simulink model "k1visitmxp"  (Simulink 8.8)
settings: Solver=ode45  StartTime=0.0  StopTime=10.0  RelTol=1e-3  EnableMultiTasking=on
libraries: cdsIPCx x26, cdsCDI64 x6, cdsCDO64 x6, BIO_CD_DECODE_MASTER x6, BIO_CD_ENCODE_MASTER x5, CHK_DIO x5, dac x3, cdsBit2Word x2, cdsAdcx0 x1, cdsAdcx1 x1, TYPEA_MASTER x1, cdsEpicsOut x1
settings Model: SuppressorTable=22 serialization::archive 11 0 3 0 0 0 11 0  Creator=controls  LastModifiedBy=controls
settings DataIOCC: SignalLoggingSaveFormat=Dataset
settings DebuggingCC: UnderspecifiedInitializationDetection=Simplified  MergeDetectMultiDrivingBlocksExec=error  FcnCallInpInsideContextMsg=error  AllowSymbolicDim=off  StateNameClashWarn=none
settings GRTTargetCC: CombineOutputUpdateFcns=on  GRTInterface=off

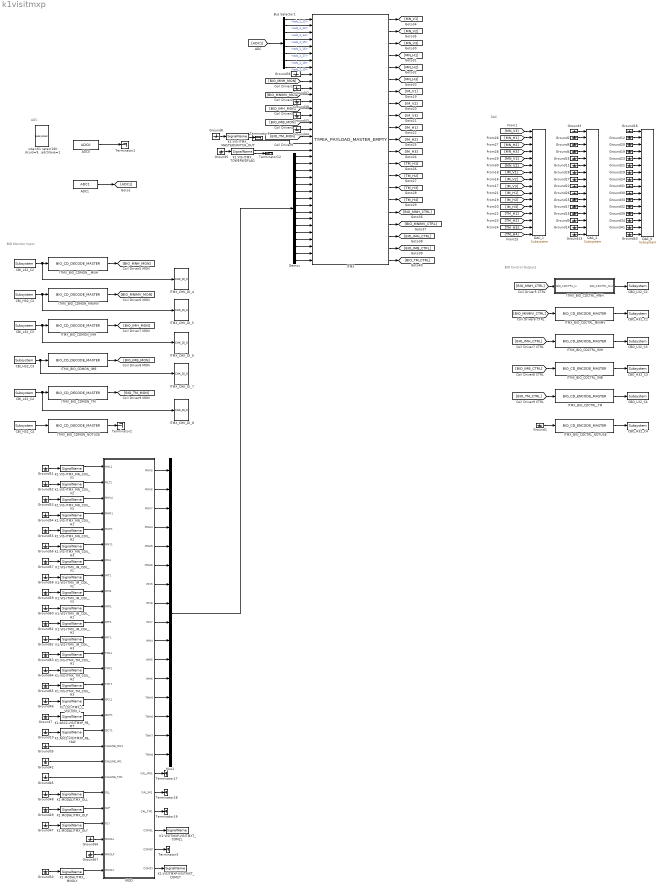
== system k1visitmxp ==
  note: BIO Monitor Input
  note: BIO Control Outputs
  note: DAC
  note: ADC
  ADC0 : cdsAdcx0/ADC0  Tag=cdsAdc  Description=|
      | type-GSC_16AI64SSA
      | card_num=0
      settings: AttributesFormatString=%<Description>\n%<Tag>
  ADC1 : cdsAdcx1/ADC1  Tag=cdsAdc  Description=|
      | type-GSC_16AI64SSA
      | card_num=1
      settings: AttributesFormatString=%<Description>\n%<Tag>
  Bus Selector1 : BusSelector  OutputSignals=adc_1_12,adc_1_13,adc_1_14,adc_1_15,adc_1_16,adc_1_17,adc_1_18,adc_1_19
  CBI_H32_C2 : cdsCDI64/Subsystem  Tag=cdsCDI64  Description=card_num=5
      settings: AttributesFormatString=%<Tag>\n%<Description>
  CBI_H32_C3 : cdsCDI64/Subsystem  Tag=cdsCDI64  Description=card_num=7
      settings: AttributesFormatString=%<Tag>\n%<Description>
  CBI_H32_C4 : cdsCDI64/Subsystem  Tag=cdsCDI64  Description=card_num=9
      settings: AttributesFormatString=%<Tag>\n%<Description>
  CBI_L32_C2 : cdsCDI64/Subsystem  Tag=cdsCDI64  Description=card_num=4
      settings: AttributesFormatString=%<Tag>\n%<Description>
  CBI_L32_C3 : cdsCDI64/Subsystem  Tag=cdsCDI64  Description=card_num=6
      settings: AttributesFormatString=%<Tag>\n%<Description>
  CBI_L32_C4 : cdsCDI64/Subsystem  Tag=cdsCDI64  Description=card_num=8
      settings: AttributesFormatString=%<Tag>\n%<Description>
  CBO_H32_C2 : cdsCDO64/Subsystem  Tag=cdsCDO64  Description=card_num=5
      settings: AttributesFormatString=%<Tag>\n%<Description>
  CBO_H32_C3 : cdsCDO64/Subsystem  Tag=cdsCDO64  Description=card_num=7
      settings: AttributesFormatString=%<Tag>\n%<Description>
  CBO_H32_C4 : cdsCDO64/Subsystem  Tag=cdsCDO64  Description=card_num=9
      settings: AttributesFormatString=%<Tag>\n%<Description>
  CBO_L32_C2 : cdsCDO64/Subsystem  Tag=cdsCDO64  Description=card_num=4
      settings: AttributesFormatString=%<Tag>\n%<Description>
  CBO_L32_C3 : cdsCDO64/Subsystem  Tag=cdsCDO64  Description=card_num=6
      settings: AttributesFormatString=%<Tag>\n%<Description>
  CBO_L32_C4 : cdsCDO64/Subsystem  Tag=cdsCDO64  Description=card_num=8
      settings: AttributesFormatString=%<Tag>\n%<Description>
  DAC_0 : dac/Subsystem  Description=|
      | type=GSC_16AO16,
      | card_num=0
      settings: AttributesFormatString=%<Description>
  DAC_1 : dac/Subsystem  Description=|
      | type=GSC_16AO16,
      | card_num=1
      settings: AttributesFormatString=%<Description>
  DAC_2 : dac/Subsystem  Description=|
      | type=GSC_16AO16,
      | card_num=2
      settings: AttributesFormatString=%<Description>
  Demux : Demux  Outputs=16
  Ground{1..67} (67 alike) : Ground
  ITMX : TYPEA_MASTER/TYPEA_PAYLOAD_MASTER_EMPTY
  ITMX_BIO_CDCTRL_IMB : BIO_CD_ENCODE_MASTER/BIO_CD_ENCODE_MASTER
  ITMX_BIO_CDCTRL_IMH : BIO_CD_ENCODE_MASTER/BIO_CD_ENCODE_MASTER
  ITMX_BIO_CDCTRL_MNH : Subsystem
  ITMX_BIO_CDCTRL_MNIMV : BIO_CD_ENCODE_MASTER/BIO_CD_ENCODE_MASTER
  ITMX_BIO_CDCTRL_NOTUSE : BIO_CD_ENCODE_MASTER/BIO_CD_ENCODE_MASTER
  ITMX_BIO_CDCTRL_TM : BIO_CD_ENCODE_MASTER/BIO_CD_ENCODE_MASTER
  ITMX_BIO_CDMON_IMB : BIO_CD_DECODE_MASTER/BIO_CD_DECODE_MASTER
  ITMX_BIO_CDMON_IMH : BIO_CD_DECODE_MASTER/BIO_CD_DECODE_MASTER
  ITMX_BIO_CDMON_MNIMV : BIO_CD_DECODE_MASTER/BIO_CD_DECODE_MASTER
  ITMX_BIO_CDMON_NOTUSE : BIO_CD_DECODE_MASTER/BIO_CD_DECODE_MASTER
  ITMX_BIO_CDMON_TM : BIO_CD_DECODE_MASTER/BIO_CD_DECODE_MASTER
  ITMX_BIO_CDMON__MNH : BIO_CD_DECODE_MASTER/BIO_CD_DECODE_MASTER
  ITMX_CHK_DI_{4..8} (5 alike) : CHK_DIO/CHK_DI_0
  K1:ASC2-VISITMXP_FB_PIT : cdsIPCx/SignalName  Tag=cdsIPCx_RFM  Description=card=0
      settings: AttributesFormatString=%<Description>\n%<Tag>
  K1:ASC2-VISITMXP_FB_YAW : cdsIPCx/SignalName  Tag=cdsIPCx_RFM  Description=card=0
      settings: AttributesFormatString=%<Description>\n%<Tag>
  K1:LSC-ITMX_L_VISITMX_L : cdsIPCx/SignalName  Tag=cdsIPCx_RFM  Description=card=0
      settings: AttributesFormatString=%<Description>\n%<Tag>
  K1:MODALITMX_MNOLY : cdsIPCx/SignalName  Tag=cdsIPCx_SHMEM  Description=Inter-Process Communication via Shared memory.
      settings: AttributesFormatString=%<Tag>
  K1:MODALITMX_OLL : cdsIPCx/SignalName  Tag=cdsIPCx_SHMEM  Description=Inter-Process Communication via Shared memory.
      settings: AttributesFormatString=%<Tag>
  K1:MODALITMX_OLP : cdsIPCx/SignalName  Tag=cdsIPCx_SHMEM  Description=Inter-Process Communication via Shared memory.
      settings: AttributesFormatString=%<Tag>
  K1:MODALITMX_OLY : cdsIPCx/SignalName  Tag=cdsIPCx_SHMEM  Description=Inter-Process Communication via Shared memory.
      settings: AttributesFormatString=%<Tag>
  K1:VIS-ITMX_IM_COIL_H1 : cdsIPCx/SignalName  Tag=cdsIPCx_SHMEM  Description=Inter-Process Communication via Shared memory.
      settings: AttributesFormatString=%<Tag>
  K1:VIS-ITMX_IM_COIL_H2 : cdsIPCx/SignalName  Tag=cdsIPCx_SHMEM  Description=Inter-Process Communication via Shared memory.
      settings: AttributesFormatString=%<Tag>
  K1:VIS-ITMX_IM_COIL_H3 : cdsIPCx/SignalName  Tag=cdsIPCx_SHMEM  Description=Inter-Process Communication via Shared memory.
      settings: AttributesFormatString=%<Tag>
  K1:VIS-ITMX_IM_COIL_V1 : cdsIPCx/SignalName  Tag=cdsIPCx_SHMEM  Description=Inter-Process Communication via Shared memory.
      settings: AttributesFormatString=%<Tag>
  K1:VIS-ITMX_IM_COIL_V2 : cdsIPCx/SignalName  Tag=cdsIPCx_SHMEM  Description=Inter-Process Communication via Shared memory.
      settings: AttributesFormatString=%<Tag>
  K1:VIS-ITMX_IM_COIL_V3 : cdsIPCx/SignalName  Tag=cdsIPCx_SHMEM  Description=Inter-Process Communication via Shared memory.
      settings: AttributesFormatString=%<Tag>
  K1:VIS-ITMX_MASTERSWITCH_OUT : cdsIPCx/SignalName  Tag=cdsIPCx_SHMEM  Description=Inter-Process Communication via Shared memory.
      settings: AttributesFormatString=%<Tag>
  K1:VIS-ITMX_MN_COIL_H1 : cdsIPCx/SignalName  Tag=cdsIPCx_SHMEM  Description=Inter-Process Communication via Shared memory.
      settings: AttributesFormatString=%<Tag>
  K1:VIS-ITMX_MN_COIL_H2 : cdsIPCx/SignalName  Tag=cdsIPCx_SHMEM  Description=Inter-Process Communication via Shared memory.
      settings: AttributesFormatString=%<Tag>
  K1:VIS-ITMX_MN_COIL_H3 : cdsIPCx/SignalName  Tag=cdsIPCx_SHMEM  Description=Inter-Process Communication via Shared memory.
      settings: AttributesFormatString=%<Tag>
  K1:VIS-ITMX_MN_COIL_V1 : cdsIPCx/SignalName  Tag=cdsIPCx_SHMEM  Description=Inter-Process Communication via Shared memory.
      settings: AttributesFormatString=%<Tag>
  K1:VIS-ITMX_MN_COIL_V2 : cdsIPCx/SignalName  Tag=cdsIPCx_SHMEM  Description=Inter-Process Communication via Shared memory.
      settings: AttributesFormatString=%<Tag>
  K1:VIS-ITMX_MN_COIL_V3 : cdsIPCx/SignalName  Tag=cdsIPCx_SHMEM  Description=Inter-Process Communication via Shared memory.
      settings: AttributesFormatString=%<Tag>
  K1:VIS-ITMX_TM_COIL_H1 : cdsIPCx/SignalName  Tag=cdsIPCx_SHMEM  Description=Inter-Process Communication via Shared memory.
      settings: AttributesFormatString=%<Tag>
  K1:VIS-ITMX_TM_COIL_H2 : cdsIPCx/SignalName  Tag=cdsIPCx_SHMEM  Description=Inter-Process Communication via Shared memory.
      settings: AttributesFormatString=%<Tag>
  K1:VIS-ITMX_TM_COIL_H3 : cdsIPCx/SignalName  Tag=cdsIPCx_SHMEM  Description=Inter-Process Communication via Shared memory.
      settings: AttributesFormatString=%<Tag>
  K1:VIS-ITMX_TOWERWDFLAG : cdsIPCx/SignalName  Tag=cdsIPCx_SHMEM  Description=Inter-Process Communication via Shared memory.
      settings: AttributesFormatString=%<Tag>
  K1:VISITMXP-VISITMXT_COM2L : cdsIPCx/SignalName  Tag=cdsIPCx_SHMEM  Description=Inter-Process Communication via Shared memory.
      settings: AttributesFormatString=%<Tag>
  K1:VISITMXP-VISITMXT_COM2Y : cdsIPCx/SignalName  Tag=cdsIPCx_SHMEM  Description=Inter-Process Communication via Shared memory.
      settings: AttributesFormatString=%<Tag>
  MOD : Subsystem  Tag=top_names
  Mux1 : Mux  Inputs=16
  Terminator{1..3,9,12,17..19} (8 alike) : Terminator
  site=K1 rate=16K dcuid=93 host=k1ix1 specific_cpu=3 adcSlave=1 : cdsParameters/Subsystem  Tag=cdsParameters  Description=|
      | Purpose:                                                                                                                                                                                                                                
      | Provide system parameters to the FE code generator to properly configure the generated EPICS names, rep rate of the FE controller, and the Data Acquisition node ID for proper storage of data from this FE controller.                 
      |                                                                                                                                                                                                                                         
      | Useage:                                                                                                                                                                                                                                 
      | The part NAME field is used to identify the FE parameters. It must be of the form:                                                                                                                                                      
      | site=                                                                                                                                                                                                                                   
      | rate=                                                                                                                                                                                                                                   
      | dcuid=                                                                                                                                                                                                                                  
      |                                                                                                                                                                                                                                         
      | Where:                                                                                                                                                                                                                                  
      | site= argument may be H1, H2, L1, M1, G1, either as a single argument or multiple, for example site=H1,H2. These are the only names allowed. These will become the first two characters of all EPICS and signal names (for example G1:).
      |                                                                                                                                                                                                                                         
      | rate= may be 2K, 16K, 32K, or 64K                                                                                                                                                                                                       
      |                                                                                                                                                                                                                                         
      | dcuid= is site specific ie it must be unique at each site.
      settings: AttributesFormatString=%<Tag>
  wires:
  ADC1/1 -> [ADC1]
  [MN_V3] -> DAC_1/1
  [MN_H1] -> DAC_1/2
  [MN_H2] -> DAC_1/3
  [MN_H3] -> DAC_1/4
  [MN_V1] -> DAC_1/5
  [MN_V2] -> DAC_1/6
  [IM_V1] -> DAC_1/7
  [IM_V2] -> DAC_1/8
  [IM_V3] -> DAC_1/9
  [IM_H1] -> DAC_1/10
  [TM_H1] -> DAC_1/13
  [TM_H4] -> DAC_1/16
  [TM_H3] -> DAC_1/15
  [TM_H2] -> DAC_1/14
  [IM_H2] -> DAC_1/11
  [IM_H3] -> DAC_1/12
  [BIO_MNH_CTRL] -> ITMX_BIO_CDCTRL_MNH/1(BIO_CDCTRL_In)
  ITMX_BIO_CDCTRL_MNH/1(DIO_CDCTRL_Out) -> CBO_L32_C2/1
  [BIO_MNIMV_CTRL] -> ITMX_BIO_CDCTRL_MNIMV/1
  ITMX_BIO_CDCTRL_MNIMV/1 -> CBO_H32_C2/1
  [BIO_IMH_CTRL] -> ITMX_BIO_CDCTRL_IMH/1
  ITMX_BIO_CDCTRL_IMH/1 -> CBO_L32_C3/1
  [BIO_IMB_CTRL] -> ITMX_BIO_CDCTRL_IMB/1
  ITMX_BIO_CDCTRL_IMB/1 -> CBO_H32_C3/1
  [BIO_TM_CTRL] -> ITMX_BIO_CDCTRL_TM/1
  ITMX_BIO_CDCTRL_TM/1 -> CBO_L32_C4/1
  Ground1/1 -> ITMX_BIO_CDCTRL_NOTUSE/1
  ITMX_BIO_CDCTRL_NOTUSE/1 -> CBO_H32_C4/1
  CBI_L32_C2/1 -> ITMX_CHK_DI_4/1, ITMX_BIO_CDMON__MNH/1
  ITMX_BIO_CDMON__MNH/1 -> [BIO_MNH_MON]
  CBI_H32_C2/1 -> ITMX_CHK_DI_5/1, ITMX_BIO_CDMON_MNIMV/1
  ITMX_BIO_CDMON_MNIMV/1 -> [BIO_MNIMV_MON]
  CBI_L32_C3/1 -> ITMX_CHK_DI_6/1, ITMX_BIO_CDMON_IMH/1
  ITMX_BIO_CDMON_IMH/1 -> [BIO_IMH_MON]
  ITMX_BIO_CDMON_IMB/1 -> [BIO_IMB_MON]
  CBI_L32_C4/1 -> ITMX_CHK_DI_8/1, ITMX_BIO_CDMON_TM/1
  ITMX_BIO_CDMON_TM/1 -> [BIO_TM_MON]
  CBI_H32_C4/1 -> ITMX_BIO_CDMON_NOTUSE/1
  ITMX_BIO_CDMON_NOTUSE/1 -> Terminator2/1
  Ground3/1 -> DAC_2/1
  Ground2/1 -> DAC_2/2
  Ground6/1 -> DAC_2/3
  Ground4/1 -> DAC_2/4
  Ground25/1 -> DAC_2/5
  Ground11/1 -> DAC_2/6
  Ground28/1 -> DAC_2/7
  Ground27/1 -> DAC_2/8
  Ground22/1 -> DAC_2/9
  Ground26/1 -> DAC_2/10
  Ground15/1 -> DAC_2/11
  Ground17/1 -> DAC_2/12
  Ground16/1 -> DAC_2/13
  Ground9/1 -> DAC_2/14
  Ground14/1 -> DAC_2/15
  Ground13/1 -> DAC_2/16
  CBI_H32_C3/1 -> ITMX_CHK_DI_7/1, ITMX_BIO_CDMON_IMB/1
  [ADC1] -> Bus Selector1/1
  K1:VIS-ITMX_TOWERWDFLAG/2 -> Terminator12/1
  Ground5/1 -> K1:VIS-ITMX_TOWERWDFLAG/1
  ADC0/1 -> Terminator1/1
  Ground18/1 -> DAC_0/1
  Ground12/1 -> DAC_0/2
  Ground19/1 -> DAC_0/4
  Ground20/1 -> DAC_0/3
  Ground29/1 -> DAC_0/7
  Ground23/1 -> DAC_0/5
  Ground21/1 -> DAC_0/6
  Ground24/1 -> DAC_0/8
  Ground31/1 -> DAC_0/9
  Ground30/1 -> DAC_0/10
  Ground33/1 -> DAC_0/11
  Ground32/1 -> DAC_0/12
  Ground39/1 -> DAC_0/13
  Ground34/1 -> DAC_0/14
  Ground41/1 -> DAC_0/15
  Ground40/1 -> DAC_0/16
  Ground8/1 -> K1:VIS-ITMX_MASTERSWITCH_OUT/1
  K1:VIS-ITMX_MASTERSWITCH_OUT/2 -> Terminator9/1
  Mux1/1 -> Demux/1
  MOD/1(MNV5) -> Mux1/1
  MOD/2(MNV6) -> Mux1/2
  MOD/3(MNV7) -> Mux1/3
  MOD/4(MNH4) -> Mux1/4
  MOD/5(MNH5) -> Mux1/5
  MOD/6(MNH6) -> Mux1/6
  MOD/7(IMV5) -> Mux1/7
  MOD/8(IMV6) -> Mux1/8
  MOD/9(IMV7) -> Mux1/9
  MOD/10(IMH4) -> Mux1/10
  MOD/11(IMH5) -> Mux1/11
  MOD/12(IMH6) -> Mux1/12
  MOD/13(TMH5) -> Mux1/13
  MOD/14(TMH6) -> Mux1/14
  MOD/15(TMH7) -> Mux1/15
  MOD/16(TMH8) -> Mux1/16
  Ground51/1 -> K1:VIS-ITMX_MN_COIL_V1/1
  Ground52/1 -> K1:VIS-ITMX_MN_COIL_V2/1
  Ground53/1 -> K1:VIS-ITMX_MN_COIL_V3/1
  Ground54/1 -> K1:VIS-ITMX_MN_COIL_H1/1
  Ground55/1 -> K1:VIS-ITMX_MN_COIL_H2/1
  Ground56/1 -> K1:VIS-ITMX_MN_COIL_H3/1
  Ground57/1 -> K1:VIS-ITMX_IM_COIL_V1/1
  Ground58/1 -> K1:VIS-ITMX_IM_COIL_V2/1
  Ground59/1 -> K1:VIS-ITMX_IM_COIL_V3/1
  Ground60/1 -> K1:VIS-ITMX_IM_COIL_H1/1
  Ground61/1 -> K1:VIS-ITMX_IM_COIL_H2/1
  Ground62/1 -> K1:VIS-ITMX_IM_COIL_H3/1
  Ground63/1 -> K1:VIS-ITMX_TM_COIL_H1/1
  Ground64/1 -> K1:VIS-ITMX_TM_COIL_H2/1
  Ground65/1 -> K1:VIS-ITMX_TM_COIL_H3/1
  K1:VIS-ITMX_MN_COIL_V1/1 -> MOD/1(MNL1)
  K1:VIS-ITMX_MN_COIL_V2/1 -> MOD/2(MLT1)
  K1:VIS-ITMX_MN_COIL_V3/1 -> MOD/3(MNV4)
  K1:VIS-ITMX_MN_COIL_H1/1 -> MOD/4(MNR1)
  K1:VIS-ITMX_MN_COIL_H2/1 -> MOD/5(MNP1)
  K1:VIS-ITMX_MN_COIL_H3/1 -> MOD/6(MNY1)
  K1:VIS-ITMX_IM_COIL_V1/1 -> MOD/7(IML1)
  K1:VIS-ITMX_IM_COIL_V2/1 -> MOD/8(IMT1)
  K1:VIS-ITMX_IM_COIL_V3/1 -> MOD/9(IMV4)
  K1:VIS-ITMX_IM_COIL_H1/1 -> MOD/10(IMR1)
  K1:VIS-ITMX_IM_COIL_H2/1 -> MOD/11(IMP1)
  K1:VIS-ITMX_IM_COIL_H3/1 -> MOD/12(IMY1)
  K1:VIS-ITMX_TM_COIL_H1/1 -> MOD/13(TML1)
  K1:VIS-ITMX_TM_COIL_H2/1 -> MOD/14(TMP1)
  K1:VIS-ITMX_TM_COIL_H3/1 -> MOD/15(TMY1)
  MOD/17(CAL_MN1) -> Terminator17/1
  MOD/18(CAL_IM1) -> Terminator18/1
  MOD/19(CAL_TM1) -> Terminator19/1
  Demux/1 -> ITMX/21
  Demux/2 -> ITMX/22
  Demux/3 -> ITMX/23
  Demux/4 -> ITMX/24
  Demux/5 -> ITMX/25
  Demux/6 -> ITMX/26
  Demux/7 -> ITMX/27
  Demux/8 -> ITMX/28
  Demux/9 -> ITMX/29
  Demux/10 -> ITMX/30
  Demux/11 -> ITMX/31
  Demux/12 -> ITMX/32
  Demux/13 -> ITMX/33
  Demux/14 -> ITMX/34
  Demux/15 -> ITMX/35
  Demux/16 -> ITMX/36
  Bus Selector1/1 -> ITMX/1  "<adc_1_12>"
  Bus Selector1/2 -> ITMX/2  "<adc_1_13>"
  Bus Selector1/3 -> ITMX/3  "<adc_1_14>"
  Bus Selector1/4 -> ITMX/4  "<adc_1_15>"
  Bus Selector1/5 -> ITMX/5  "<adc_1_16>"
  Bus Selector1/6 -> ITMX/6  "<adc_1_17>"
  Bus Selector1/7 -> ITMX/7  "<adc_1_18>"
  Bus Selector1/8 -> ITMX/8  "<adc_1_19>"
  [BIO_IMH_MON] -> ITMX/14
  Ground38/1 -> ITMX/13
  Ground36/1 -> ITMX/9
  Ground37/1 -> ITMX/11
  [BIO_MNH_MON] -> ITMX/10
  [BIO_MNIMV_MON] -> ITMX/12
  [BIO_IMB_MON] -> ITMX/16
  [BIO_TM_MON] -> ITMX/18
  Ground44/1 -> ITMX/17
  Ground43/1 -> ITMX/15
  K1:VIS-ITMX_TOWERWDFLAG/1 -> ITMX/20
  K1:VIS-ITMX_MASTERSWITCH_OUT/1 -> ITMX/19
  ITMX/1 -> [MN_V1]
  ITMX/2 -> [MN_V2]
  ITMX/3 -> [MN_V3]
  ITMX/4 -> [MN_H1]
  ITMX/5 -> [MN_H2]
  ITMX/6 -> [MN_H3]
  ITMX/7 -> [IM_V1]
  ITMX/8 -> [IM_V2]
  ITMX/9 -> [IM_V3]
  ITMX/10 -> [IM_H1]
  ITMX/11 -> [IM_H2]
  ITMX/12 -> [IM_H3]
  ITMX/13 -> [TM_H1]
  ITMX/14 -> [TM_H2]
  ITMX/15 -> [TM_H3]
  ITMX/16 -> [TM_H4]
  ITMX/17 -> [BIO_MNH_CTRL]
  ITMX/18 -> [BIO_MNIMV_CTRL]
  ITMX/19 -> [BIO_IMH_CTRL]
  ITMX/20 -> [BIO_IMB_CTRL]
  ITMX/21 -> [BIO_TM_CTRL]
  K1:ASC2-VISITMXP_FB_PIT/1 -> MOD/17(ISCP1)
  K1:ASC2-VISITMXP_FB_YAW/1 -> MOD/18(ISCY1)
  Ground7/1 -> K1:ASC2-VISITMXP_FB_PIT/1
  Ground10/1 -> K1:ASC2-VISITMXP_FB_YAW/1
  Ground35/1 -> MOD/19(CALLINE_MN1)
  Ground42/1 -> MOD/20(CALLINE_IM1)
  Ground45/1 -> MOD/21(CALLINE_TM1)
  K1:LSC-ITMX_L_VISITMX_L/1 -> MOD/16(ISCL1)
  Ground46/1 -> K1:LSC-ITMX_L_VISITMX_L/1
  MOD/20(COM3L) -> K1:VISITMXP-VISITMXT_COM2L/1
  MOD/22(COM3Y) -> K1:VISITMXP-VISITMXT_COM2Y/1
  MOD/21(COM3P) -> Terminator3/1
  K1:MODALITMX_OLL/1 -> MOD/22(OLL)
  K1:MODALITMX_OLP/1 -> MOD/23(OLP)
  K1:MODALITMX_OLY/1 -> MOD/24(OLY)
  Ground49/1 -> K1:MODALITMX_OLP/1
  Ground47/1 -> K1:MODALITMX_OLY/1
  Ground48/1 -> K1:MODALITMX_OLL/1
  Ground67/1 -> MOD/26(MNOLP)
  Ground66/1 -> MOD/25(MNOLL)
  Ground50/1 -> K1:MODALITMX_MNOLY/1
  K1:MODALITMX_MNOLY/1 -> MOD/27(MNOLY)

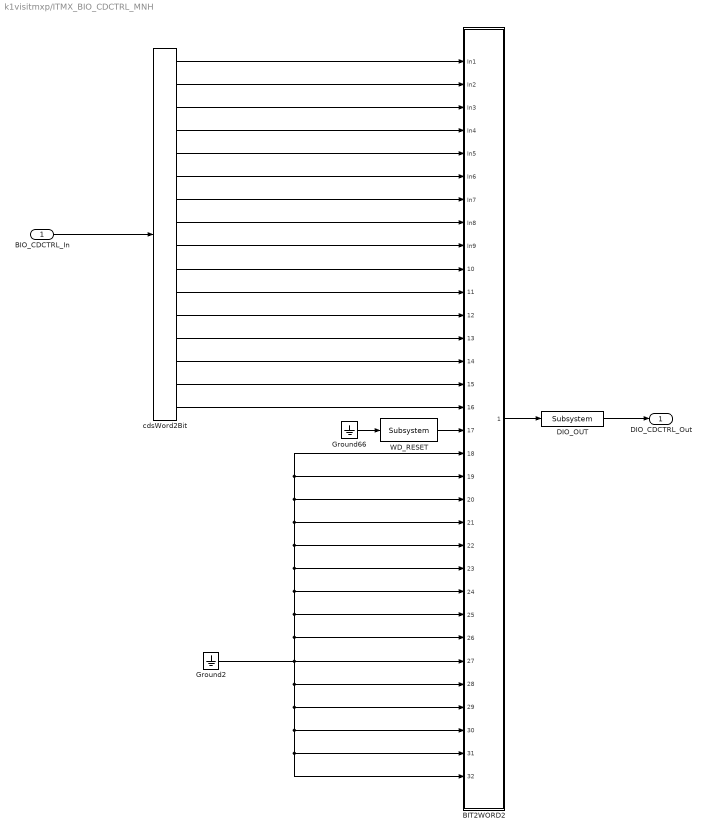
== system k1visitmxp/ITMX_BIO_CDCTRL_MNH ==
  BIO_CDCTRL_In : Inport
  BIT2WORD2 : Subsystem
  DIO_OUT : cdsEpicsOut/Subsystem  Tag=cdsEpicsOutput  Description=|
      | Purpose:                                          
      | Output a FE signal to an EPICS channel.           
      |                                                   
      | Operation:                                        
      | Takes input value and passes it to EPICS record.  
      |                                                   
      | Usage:                                            
      | Name the part with the desired EPICS rrecord name.
      settings: AttributesFormatString=%<Tag>
  Ground2 : Ground
  Ground66 : Ground
  WD_RESET : cdsEpicsBinIn/Subsystem  Tag=cdsEpicsBinIn  Description=|
      | Purpose:                                                                            
      | Create an EPICS binary (0 or 1) input channel to the FE realtime controls.          
      |                                                                                     
      | Operation:                                                                          
      | Outputs value from an EPICS ai record. Value is binary input (bi Epics record type).
      |                                                                                     
      | Usage:                                                                              
      | Name the part with the desired EPICS channel name.
      settings: AttributesFormatString=%<Tag>
  cdsWord2Bit : cdsWord2Bit/cdsWord2Bit  Tag=cdsWord2Bit  Description=Generate 16 0/1 outputs from single 16-bit integer input
      settings: AttributesFormatString=cdsWord2Bit
  DIO_CDCTRL_Out : Outport
  wires:
  BIT2WORD2/1(Out1) -> DIO_OUT/1
  DIO_OUT/1 -> DIO_CDCTRL_Out/1
  BIO_CDCTRL_In/1 -> cdsWord2Bit/1
  cdsWord2Bit/1 -> BIT2WORD2/1(In1)
  cdsWord2Bit/2 -> BIT2WORD2/2(In2)
  cdsWord2Bit/3 -> BIT2WORD2/3(In3)
  cdsWord2Bit/4 -> BIT2WORD2/4(In4)
  cdsWord2Bit/5 -> BIT2WORD2/5(In5)
  cdsWord2Bit/6 -> BIT2WORD2/6(In6)
  cdsWord2Bit/7 -> BIT2WORD2/7(In7)
  cdsWord2Bit/8 -> BIT2WORD2/8(In8)
  cdsWord2Bit/9 -> BIT2WORD2/9(In9)
  cdsWord2Bit/10 -> BIT2WORD2/10(In10)
  cdsWord2Bit/11 -> BIT2WORD2/11(In11)
  cdsWord2Bit/12 -> BIT2WORD2/12(In12)
  cdsWord2Bit/13 -> BIT2WORD2/13(In13)
  cdsWord2Bit/14 -> BIT2WORD2/14(In14)
  cdsWord2Bit/15 -> BIT2WORD2/15(In15)
  cdsWord2Bit/16 -> BIT2WORD2/16(In16)
  WD_RESET/1 -> BIT2WORD2/17(In17)
  Ground66/1 -> WD_RESET/1
  Ground2/1 -> BIT2WORD2/27(In27), BIT2WORD2/28(In28), BIT2WORD2/29(In29), BIT2WORD2/30(In30), BIT2WORD2/31(In31), BIT2WORD2/32(In32), BIT2WORD2/26(In26), BIT2WORD2/25(In25), BIT2WORD2/24(In24), BIT2WORD2/23(In23), BIT2WORD2/22(In22), BIT2WORD2/21(In21), BIT2WORD2/20(In20), BIT2WORD2/18(In18), BIT2WORD2/19(In19)

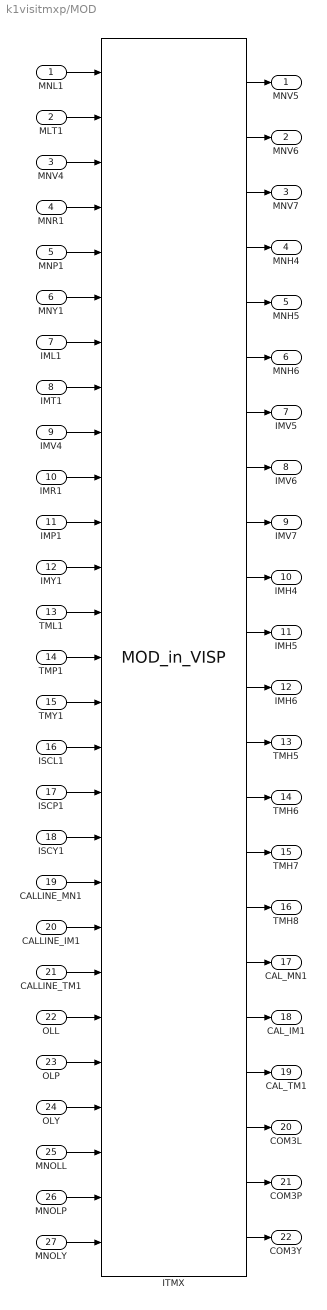
== system k1visitmxp/MOD ==
  MNL1 : Inport
  MLT1 : Inport  Port=2
  MNV4 : Inport  Port=3
  MNR1 : Inport  Port=4
  MNP1 : Inport  Port=5
  MNY1 : Inport  Port=6
  IML1 : Inport  Port=7
  IMT1 : Inport  Port=8
  IMV4 : Inport  Port=9
  IMR1 : Inport  Port=10
  IMP1 : Inport  Port=11
  IMY1 : Inport  Port=12
  TML1 : Inport  Port=13
  TMP1 : Inport  Port=14
  TMY1 : Inport  Port=15
  ISCL1 : Inport  Port=16
  ISCP1 : Inport  Port=17
  ISCY1 : Inport  Port=18
  CALLINE_MN1 : Inport  Port=19
  CALLINE_IM1 : Inport  Port=20
  CALLINE_TM1 : Inport  Port=21
  OLL : Inport  Port=22
  OLP : Inport  Port=23
  OLY : Inport  Port=24
  MNOLL : Inport  Port=25
  MNOLP : Inport  Port=26
  MNOLY : Inport  Port=27
  ITMX : VIS_LIB/MODAL/MOD_in_VISP  Tag=top_names
  MNV5 : Outport
  MNV6 : Outport  Port=2
  MNV7 : Outport  Port=3
  MNH4 : Outport  Port=4
  MNH5 : Outport  Port=5
  MNH6 : Outport  Port=6
  IMV5 : Outport  Port=7
  IMV6 : Outport  Port=8
  IMV7 : Outport  Port=9
  IMH4 : Outport  Port=10
  IMH5 : Outport  Port=11
  IMH6 : Outport  Port=12
  TMH5 : Outport  Port=13
  TMH6 : Outport  Port=14
  TMH7 : Outport  Port=15
  TMH8 : Outport  Port=16
  CAL_MN1 : Outport  Port=17
  CAL_IM1 : Outport  Port=18
  CAL_TM1 : Outport  Port=19
  COM3L : Outport  Port=20
  COM3P : Outport  Port=21
  COM3Y : Outport  Port=22
  wires:
  MNL1/1 -> ITMX/1
  TMY1/1 -> ITMX/15
  MLT1/1 -> ITMX/2
  MNV4/1 -> ITMX/3
  MNR1/1 -> ITMX/4
  MNP1/1 -> ITMX/5
  MNY1/1 -> ITMX/6
  IML1/1 -> ITMX/7
  IMT1/1 -> ITMX/8
  IMV4/1 -> ITMX/9
  IMR1/1 -> ITMX/10
  IMP1/1 -> ITMX/11
  IMY1/1 -> ITMX/12
  TML1/1 -> ITMX/13
  TMP1/1 -> ITMX/14
  ITMX/1 -> MNV5/1
  ITMX/16 -> TMH8/1
  ITMX/2 -> MNV6/1
  ITMX/3 -> MNV7/1
  ITMX/4 -> MNH4/1
  ITMX/5 -> MNH5/1
  ITMX/6 -> MNH6/1
  ITMX/7 -> IMV5/1
  ITMX/8 -> IMV6/1
  ITMX/9 -> IMV7/1
  ITMX/10 -> IMH4/1
  ITMX/11 -> IMH5/1
  ITMX/12 -> IMH6/1
  ITMX/13 -> TMH5/1
  ITMX/14 -> TMH6/1
  ITMX/15 -> TMH7/1
  ISCL1/1 -> ITMX/16
  CALLINE_TM1/1 -> ITMX/21
  CALLINE_IM1/1 -> ITMX/20
  CALLINE_MN1/1 -> ITMX/19
  ISCP1/1 -> ITMX/17
  ISCY1/1 -> ITMX/18
  ITMX/17 -> CAL_MN1/1
  ITMX/18 -> CAL_IM1/1
  ITMX/19 -> CAL_TM1/1
  ITMX/20 -> COM3L/1
  ITMX/22 -> COM3Y/1
  ITMX/21 -> COM3P/1
  OLY/1 -> ITMX/24
  OLP/1 -> ITMX/23
  OLL/1 -> ITMX/22
  MNOLY/1 -> ITMX/27
  MNOLP/1 -> ITMX/26
  MNOLL/1 -> ITMX/25

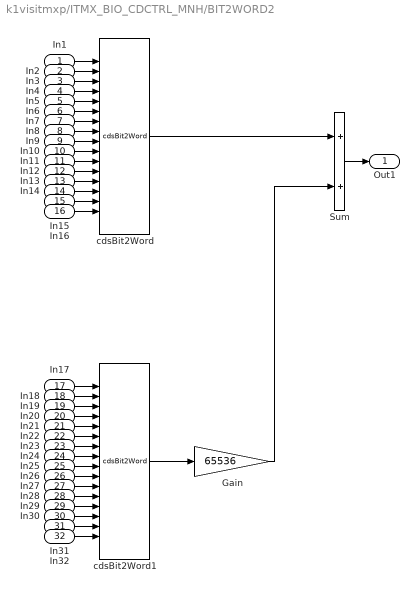
== system k1visitmxp/ITMX_BIO_CDCTRL_MNH/BIT2WORD2 ==
  In1 : Inport
  In2 : Inport  Port=2
  In3 : Inport  Port=3
  In4 : Inport  Port=4
  In5 : Inport  Port=5
  In6 : Inport  Port=6
  In7 : Inport  Port=7
  In8 : Inport  Port=8
  In9 : Inport  Port=9
  In10 : Inport  Port=10
  In11 : Inport  Port=11
  In12 : Inport  Port=12
  In13 : Inport  Port=13
  In14 : Inport  Port=14
  In15 : Inport  Port=15
  In16 : Inport  Port=16
  In17 : Inport  Port=17
  In18 : Inport  Port=18
  In19 : Inport  Port=19
  In20 : Inport  Port=20
  In21 : Inport  Port=21
  In22 : Inport  Port=22
  In23 : Inport  Port=23
  In24 : Inport  Port=24
  In25 : Inport  Port=25
  In26 : Inport  Port=26
  In27 : Inport  Port=27
  In28 : Inport  Port=28
  In29 : Inport  Port=29
  In30 : Inport  Port=30
  In31 : Inport  Port=31
  In32 : Inport  Port=32
  Gain : Gain  Gain=65536
  Sum : Sum
  cdsBit2Word : cdsBit2Word/cdsBit2Word  Tag=cdsBit2Word  Description=Forms single 16 bit integer from 16 0/1 inputs.
      settings: AttributesFormatString=%<Tag>
  cdsBit2Word1 : cdsBit2Word/cdsBit2Word  Tag=cdsBit2Word  Description=Forms single 16 bit integer from 16 0/1 inputs.
      settings: AttributesFormatString=%<Tag>
  Out1 : Outport
  wires:
  In32/1 -> cdsBit2Word1/16
  In31/1 -> cdsBit2Word1/15
  In30/1 -> cdsBit2Word1/14
  In29/1 -> cdsBit2Word1/13
  In28/1 -> cdsBit2Word1/12
  In27/1 -> cdsBit2Word1/11
  In26/1 -> cdsBit2Word1/10
  In25/1 -> cdsBit2Word1/9
  In24/1 -> cdsBit2Word1/8
  In23/1 -> cdsBit2Word1/7
  In22/1 -> cdsBit2Word1/6
  In21/1 -> cdsBit2Word1/5
  In20/1 -> cdsBit2Word1/4
  In19/1 -> cdsBit2Word1/3
  In18/1 -> cdsBit2Word1/2
  In17/1 -> cdsBit2Word1/1
  In16/1 -> cdsBit2Word/16
  In15/1 -> cdsBit2Word/15
  In14/1 -> cdsBit2Word/14
  In13/1 -> cdsBit2Word/13
  In12/1 -> cdsBit2Word/12
  In11/1 -> cdsBit2Word/11
  Sum/1 -> Out1/1
  In10/1 -> cdsBit2Word/10
  In9/1 -> cdsBit2Word/9
  In8/1 -> cdsBit2Word/8
  In7/1 -> cdsBit2Word/7
  In6/1 -> cdsBit2Word/6
  In5/1 -> cdsBit2Word/5
  In4/1 -> cdsBit2Word/4
  In3/1 -> cdsBit2Word/3
  In2/1 -> cdsBit2Word/2
  In1/1 -> cdsBit2Word/1
  cdsBit2Word/1 -> Sum/1
  cdsBit2Word1/1 -> Gain/1
  Gain/1 -> Sum/2
